simulink model "PI"  (R2021a)
settings: Solver=FixedStepAuto  StartTime=0.0  StopTime=Inf  FixedStep=0.01  RelTol=1e-3  EnableMultiTasking=on
undefined symbols (not defined in the file): DiscIntNeverNeededParam
libraries: arduinolib x4, simulink x1
settings Model: SILPILModeSetting=veronly  ExtModeTrigDuration=2  Creator=Simón  LastModifiedBy=Simón
settings OptimizationCC: EnhancedBackFolding=on  PassReuseOutputArgsAs=Individual arguments  ZeroExternalMemoryAtStartup=off  ZeroInternalMemoryAtStartup=off  MaxStackSize=64  OptimizeBlockOrder=speed  DifferentSizesBufferReuse=on  OptimizationCustomize=off  EfficientTunableParamExpr=on
settings DebuggingCC: ParameterTunabilityLossMsg=error
settings HardwareCC: ProdBitPerInt=16  ProdBitPerPointer=16  ProdBitPerSizeT=16  ProdBitPerPtrDiffT=16  ProdLargestAtomicFloat=None  ProdWordSize=8  ProdHWDeviceType=Atmel->AVR  UseEmbeddedCoderFeatures=off  UseSimulinkCoderFeatures=off
settings SFSimCC: MATLABDynamicMemAlloc=off
settings RTWCC: SystemTargetFile=ert.tlc  HardwareBoard=Arduino Uno  TemplateMakefile=ert_default_tmf  Toolchain=Arduino AVR  BuildConfiguration=Faster Runs
settings CodeAppCC: ForceParamTrailComments=on  IgnoreCustomStorageClasses=off  OperatorAnnotations=on  SimulinkDataObjDesc=on  SFDataObjDesc=on  InsertBlockDesc=on
settings ERTTargetCC: SupportContinuousTime=on  SupportNonInlinedSFcns=on  SupportVariableSizeSignals=on  ExtModeStaticAllocSize=250

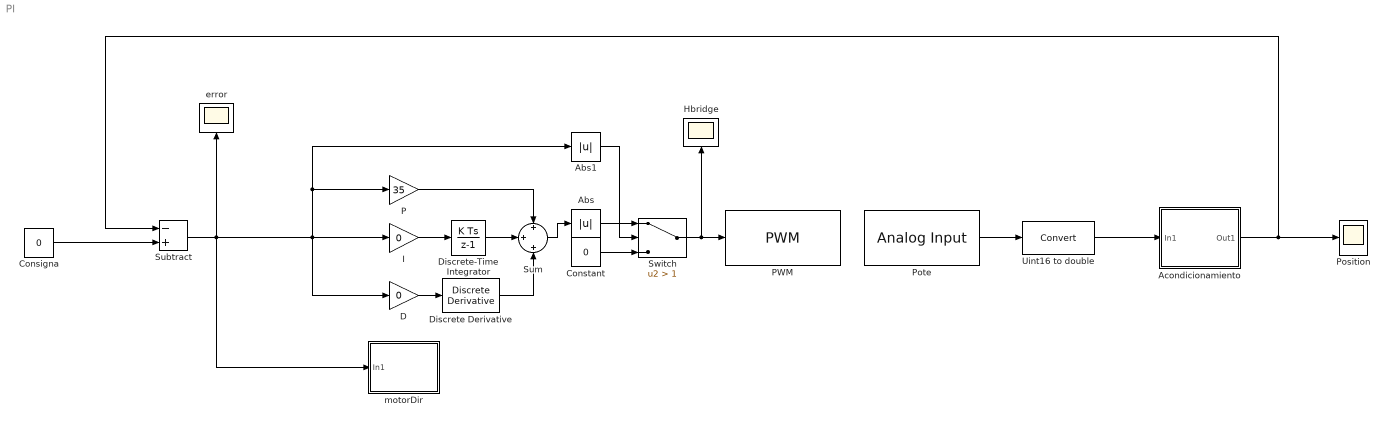
== system PI ==
  Abs : Abs
  Abs1 : Abs
  Acondicionamiento : Subsystem
  Consigna : Constant  Value=0
  Constant : Constant  Value=0
  D : Gain  Gain=0
  Discrete Derivative : simulink/Discrete/Discrete Derivative  gainval=1.0  ICPrevScaledInput=0.0  OutMin=[]  OutMax=[]  OutDataType=fixdt(1, 16)  OutScaling=2^-10  DoSatur=off
  Discrete-Time Integrator : DiscreteIntegrator  SampleTime=-1  ICPrevOutput=DiscIntNeverNeededParam  ICPrevScaledInput=DiscIntNeverNeededParam
  Hbridge : Scope
  I : Gain  Gain=0
  P : Gain  Gain=35
  PWM : arduinolib/PWM  pinNumber=10  frequencyType=Default  desiredFrequency=490.2  achievableFrequency=490.2
  Position : Scope
  Pote : arduinolib/Analog Input  pinNumber=0  ReadResultsOnly=off  ConversionTriggerSource=Software  ExternalTriggerType=uint32( 0 )  OutputDataType=uint16  EnableConversionCompleteNotify=off  EnableOuputStatus=off  SampleTime=-1  blockPlatform=arduino
  Subtract : Sum  Inputs=-+
  Sum : Sum  Inputs=+|+|+
  Switch : Switch  Criteria=u2 > Threshold  Threshold=1
  Uint16 to double : DataTypeConversion
  error : Scope
  motorDir : Subsystem
  wires:
  Pote/1 -> Uint16 to double/1
  Uint16 to double/1 -> Acondicionamiento/1(In1)
  Consigna/1 -> Subtract/2
  Sum/1 -> Abs/1
  Discrete-Time Integrator/1 -> Sum/2
  I/1 -> Discrete-Time Integrator/1
  P/1 -> Sum/1
  Acondicionamiento/1(Out1) -> Subtract/1, Position/1
  Constant/1 -> Switch/3
  Abs1/1 -> Switch/2
  Subtract/1 -> D/1, Abs1/1, P/1, I/1, motorDir/1(In1), error/1
  Abs/1 -> Switch/1
  Switch/1 -> Hbridge/1, PWM/1
  D/1 -> Discrete Derivative/1
  Discrete Derivative/1 -> Sum/3

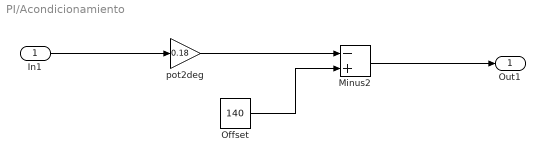
== system PI/Acondicionamiento ==
  In1 : Inport
  Minus2 : Sum  Inputs=-+
  Offset : Constant  Value=140
  pot2deg : Gain  Gain=0.18
  Out1 : Outport
  wires:
  Offset/1 -> Minus2/2
  pot2deg/1 -> Minus2/1
  Minus2/1 -> Out1/1
  In1/1 -> pot2deg/1

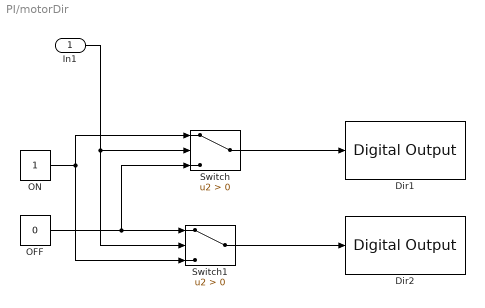
== system PI/motorDir ==
  In1 : Inport
  Dir1 : arduinolib/Digital Output  pinNumber=8  Direction=output  blockPlatform=arduino
  Dir2 : arduinolib/Digital Output  pinNumber=9  Direction=output  blockPlatform=arduino
  OFF : Constant  Value=0
  ON : Constant
  Switch : Switch  Criteria=u2 > Threshold
  Switch1 : Switch  Criteria=u2 > Threshold
  wires:
  In1/1 -> Switch1/2, Switch/2
  OFF/1 -> Switch/3, Switch1/1
  ON/1 -> Switch1/3, Switch/1
  Switch1/1 -> Dir2/1
  Switch/1 -> Dir1/1
